simulink model "control_on_off"  (R2020b)
settings: Solver=VariableStepAuto  StartTime=0.0  StopTime=10.0  RelTol=1e-3
settings Model: Creator=Acer  LastModifiedBy=Acer

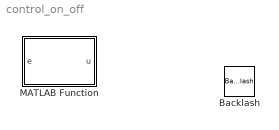
== system control_on_off ==
  Backlash : Backlash
  MATLAB Function : MATLAB Function  TreatAsAtomicUnit=on

== matlab function control_on_off/MATLAB Function ==
  data: e input; u output
function u = control_on_off(e)
if (e>=0)
    u=1;
end

if e<0
    u=0;
end
